simulink model "try1"  (R2021a)
settings: Solver=VariableStepAuto  StartTime=0.0  StopTime=10.0  RelTol=1e-3
libraries: spsDiodeLib x4, spsSeriesRLCBranchLib x2, spsACVoltageSourceLib x1, spsVoltageMeasurementLib x1
settings Model: Creator=Ahmed  LastModifiedBy=Ahmed

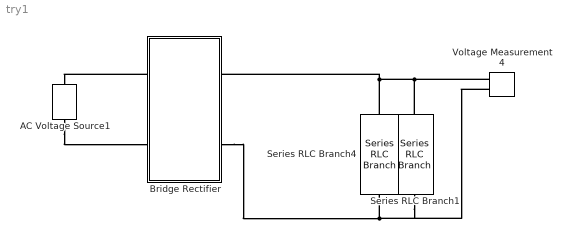
== system try1 ==
  AC Voltage Source1 : spsACVoltageSourceLib/AC Voltage Source  Amplitude=220*sqrt(2)  Phase=0  Frequency=50  SampleTime=0  Measurements=None  BusType=swing  Pref=10e3  Qref=0  Qmin=-inf  Qmax=+inf
  Bridge Rectifier : Subsystem
  Series RLC Branch1 : spsSeriesRLCBranchLib/Series RLC Branch  LConnTagsString=__new0  RConnTagsString=__new0  BranchType=R  Resistance=1e03  Inductance=1e-3  SetiL0=off  InitialCurrent=0  Capacitance=100e-6  Setx0=off  InitialVoltage=0  Measurements=None
  Series RLC Branch4 : spsSeriesRLCBranchLib/Series RLC Branch  LConnTagsString=__new0  RConnTagsString=__new0  BranchType=C  Resistance=1  Inductance=1e-3  SetiL0=off  InitialCurrent=0  Capacitance=100e-6  Setx0=off  InitialVoltage=0  Measurements=None
  Voltage Measurement4 : spsVoltageMeasurementLib/Voltage Measurement  PhasorSimulation=off  OutputType=Complex  PSBequivalent=0
  connections:
  AC Voltage Source1/LConn1 -- Bridge Rectifier/LConn2
  Bridge Rectifier/LConn1 -- AC Voltage Source1/RConn1
  Bridge Rectifier/RConn2 -- Voltage Measurement4/LConn2 -- Series RLC Branch1/RConn1 -- Series RLC Branch4/RConn1
  Voltage Measurement4/LConn1 -- Series RLC Branch1/LConn1 -- Bridge Rectifier/RConn1 -- Series RLC Branch4/LConn1

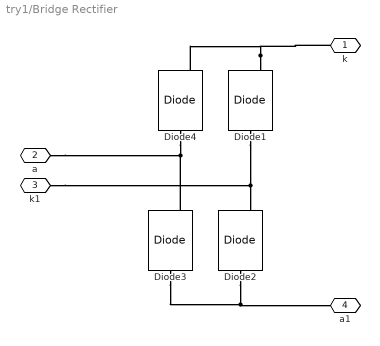
== system try1/Bridge Rectifier ==
  Diode{1..4} (4 alike) : spsDiodeLib/Diode  Ron=0.001  Lon=0  Vf=0.7  IC=0  UseSnubber=0  Rs=500  Cs=250e-9  Measurements=on
  k : PMIOPort  Side=Right
  a : PMIOPort  Port=2  Side=Left
  k1 : PMIOPort  Port=3  Side=Left
  a1 : PMIOPort  Port=4  Side=Right
  connections:
  Diode1/LConn1 -- k1/RConn1 -- Diode2/RConn1
  Diode1/RConn1 -- Diode4/RConn1 -- k/RConn1
  Diode3/RConn1 -- Diode4/LConn1 -- a/RConn1
  Diode2/LConn1 -- a1/RConn1 -- Diode3/LConn1
